simulink model "fourteen_bus_partial_linear"  (R2020b)
settings: Solver=VariableStepAuto  StartTime=0.0  StopTime=1  RelTol=1e-3
libraries: powerlib x95, powerlib_meascontrol x2
(part 2 of 2)

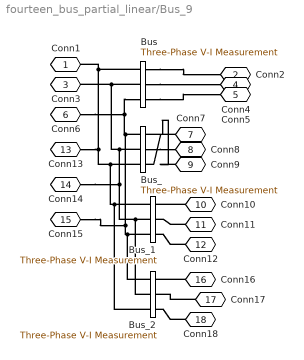
== system fourteen_bus_partial_linear/Bus_9 ==
  Bus : powerlib/Measurements/Three-Phase V-I Measurement  VoltageMeasurement=phase-to-phase  SetLabelV=on  LabelV=VB_9  Vpu=off  VpuLL=off  CurrentMeasurement=yes  SetLabelI=on  LabelI=IB_9  Ipu=off  Pbase=100e6  Vbase=500e3  OutputType=Complex  PhasorSimulation=off  PSBequivalent=0
  Bus_ : powerlib/Measurements/Three-Phase V-I Measurement  VoltageMeasurement=phase-to-phase  SetLabelV=on  LabelV=V_B9_9  Vpu=off  VpuLL=off  CurrentMeasurement=yes  SetLabelI=on  LabelI=I_B9_9  Ipu=off  Pbase=100e6  Vbase=500e3  OutputType=Complex  PhasorSimulation=off  PSBequivalent=0
  Bus_1 : powerlib/Measurements/Three-Phase V-I Measurement  VoltageMeasurement=phase-to-phase  SetLabelV=on  LabelV=V_B9  Vpu=off  VpuLL=off  CurrentMeasurement=yes  SetLabelI=on  LabelI=I_B9  Ipu=off  Pbase=100e6  Vbase=500e3  OutputType=Complex  PhasorSimulation=off  PSBequivalent=0
  Bus_2 : powerlib/Measurements/Three-Phase V-I Measurement  VoltageMeasurement=phase-to-phase  SetLabelV=on  LabelV=V_B9__9  Vpu=off  VpuLL=off  CurrentMeasurement=yes  SetLabelI=on  LabelI=I_B9__9  Ipu=off  Pbase=100e6  Vbase=500e3  OutputType=Complex  PhasorSimulation=off  PSBequivalent=0
  Conn1 : PMIOPort  Side=Left
  Conn2 : PMIOPort  Port=2  Side=Right
  Conn3 : PMIOPort  Port=3  Side=Left
  Conn4 : PMIOPort  Port=4  Side=Right
  Conn5 : PMIOPort  Port=5  Side=Right
  Conn6 : PMIOPort  Port=6  Side=Left
  Conn7 : PMIOPort  Port=7  Side=Right
  Conn8 : PMIOPort  Port=8  Side=Right
  Conn9 : PMIOPort  Port=9  Side=Right
  Conn10 : PMIOPort  Port=10  Side=Right
  Conn11 : PMIOPort  Port=11  Side=Right
  Conn12 : PMIOPort  Port=12  Side=Right
  Conn13 : PMIOPort  Port=13  Side=Left
  Conn14 : PMIOPort  Port=14  Side=Left
  Conn15 : PMIOPort  Port=15  Side=Left
  Conn16 : PMIOPort  Port=16  Side=Right
  Conn17 : PMIOPort  Port=17  Side=Right
  Conn18 : PMIOPort  Port=18  Side=Right
  connections:
  Bus/LConn1 -- Conn1/RConn1 -- Conn13/RConn1 -- Bus_/LConn3 -- Bus_1/LConn1 -- Bus_2/LConn3
  Conn3/RConn1 -- Bus/LConn2 -- Bus_/LConn2 -- Conn14/RConn1 -- Bus_1/LConn2 -- Bus_2/LConn2
  Bus_/RConn2 -- Conn8/RConn1
  Bus/RConn2 -- Conn4/RConn1
  Bus/LConn3 -- Conn6/RConn1 -- Bus_/LConn1 -- Conn15/RConn1 -- Bus_1/LConn3 -- Bus_2/LConn1
  Bus/RConn1 -- Conn2/RConn1
  Bus/RConn3 -- Conn5/RConn1
  Conn10/RConn1 -- Bus_1/RConn1
  Conn11/RConn1 -- Bus_1/RConn2
  Conn12/RConn1 -- Bus_1/RConn3
  Conn16/RConn1 -- Bus_2/RConn1
  Conn17/RConn1 -- Bus_2/RConn2
  Conn18/RConn1 -- Bus_2/RConn3
  Conn7/RConn1 -- Bus_/RConn3
  Conn9/RConn1 -- Bus_/RConn1

== system fourteen_bus_partial_linear/Subsystem ==
  Ia : Inport
  Ib : Inport  Port=2
  Ic : Inport  Port=3
  Controlled Current Source10 : powerlib/Electrical Sources/Controlled Current Source  Initialize=on  Source_Type=AC  Amplitude=0  Phase=0  Frequency=0  Measurements=None
  Controlled Current Source11 : powerlib/Electrical Sources/Controlled Current Source  Initialize=on  Source_Type=AC  Amplitude=0  Phase=0  Frequency=0  Measurements=None
  Controlled Current Source9 : powerlib/Electrical Sources/Controlled Current Source  Initialize=on  Source_Type=AC  Amplitude=0  Phase=0  Frequency=0  Measurements=None
  Ground2 : powerlib/Elements/Ground  LConnTagsString=a
  A : PMIOPort  Side=Right
  B : PMIOPort  Port=2  Side=Right
  C : PMIOPort  Port=3  Side=Right
  wires:
  Ia/1 -> Controlled Current Source9/1
  Ic/1 -> Controlled Current Source11/1
  Ib/1 -> Controlled Current Source10/1
  connections:
  Controlled Current Source10/RConn1 -- B/RConn1
  Controlled Current Source9/RConn1 -- A/RConn1
  Controlled Current Source11/RConn1 -- C/RConn1
  Controlled Current Source11/LConn1 -- Controlled Current Source9/LConn1 -- Controlled Current Source10/LConn1 -- Ground2/LConn1

== system fourteen_bus_partial_linear/Subsystem10 ==
  From Workspace15 : FromWorkspace  VariableName=load5_Ia_ts
  From Workspace16 : FromWorkspace  VariableName=load5_Ib_ts
  From Workspace17 : FromWorkspace  VariableName=load5_Ic_ts
  Subsystem3 : Subsystem
  A : PMIOPort  Side=Right
  B : PMIOPort  Port=2  Side=Right
  C : PMIOPort  Port=3  Side=Right
  wires:
  From Workspace15/1 -> Subsystem3/1(Ia)
  From Workspace17/1 -> Subsystem3/3(Ic)
  From Workspace16/1 -> Subsystem3/2(Ib)
  connections:
  Subsystem3/RConn2 -- B/RConn1
  Subsystem3/RConn1 -- A/RConn1
  Subsystem3/RConn3 -- C/RConn1

== system fourteen_bus_partial_linear/Subsystem11 ==
  From Workspace15 : FromWorkspace  VariableName=load2_Ia_ts
  From Workspace16 : FromWorkspace  VariableName=load2_Ib_ts
  From Workspace17 : FromWorkspace  VariableName=load2_Ic_ts
  Subsystem3 : Subsystem
  A : PMIOPort  Side=Right
  B : PMIOPort  Port=2  Side=Right
  C : PMIOPort  Port=3  Side=Right
  wires:
  From Workspace15/1 -> Subsystem3/1(Ia)
  From Workspace17/1 -> Subsystem3/3(Ic)
  From Workspace16/1 -> Subsystem3/2(Ib)
  connections:
  Subsystem3/RConn2 -- B/RConn1
  Subsystem3/RConn1 -- A/RConn1
  Subsystem3/RConn3 -- C/RConn1

== system fourteen_bus_partial_linear/Subsystem12 ==
  From Workspace10 : FromWorkspace  VariableName=sc3_Ib_ts
  From Workspace11 : FromWorkspace  VariableName=sc3_Ic_ts
  From Workspace9 : FromWorkspace  VariableName=sc3_Ia_ts
  Subsystem1 : Subsystem
  A : PMIOPort  Side=Right
  B : PMIOPort  Port=2  Side=Right
  C : PMIOPort  Port=3  Side=Right
  wires:
  From Workspace11/1 -> Subsystem1/3(Ic)
  From Workspace9/1 -> Subsystem1/1(Ia)
  From Workspace10/1 -> Subsystem1/2(Ib)
  connections:
  Subsystem1/RConn1 -- A/RConn1
  Subsystem1/RConn2 -- B/RConn1
  Subsystem1/RConn3 -- C/RConn1

== system fourteen_bus_partial_linear/Subsystem10/Subsystem3 ==
  Ia : Inport
  Ib : Inport  Port=2
  Ic : Inport  Port=3
  Controlled Current Source10 : powerlib/Electrical Sources/Controlled Current Source  Initialize=on  Source_Type=AC  Amplitude=0  Phase=0  Frequency=0  Measurements=None
  Controlled Current Source11 : powerlib/Electrical Sources/Controlled Current Source  Initialize=on  Source_Type=AC  Amplitude=0  Phase=0  Frequency=0  Measurements=None
  Controlled Current Source9 : powerlib/Electrical Sources/Controlled Current Source  Initialize=on  Source_Type=AC  Amplitude=0  Phase=0  Frequency=0  Measurements=None
  Ground2 : powerlib/Elements/Ground  LConnTagsString=a
  A : PMIOPort  Side=Right
  B : PMIOPort  Port=2  Side=Right
  C : PMIOPort  Port=3  Side=Right
  wires:
  Ia/1 -> Controlled Current Source9/1
  Ic/1 -> Controlled Current Source11/1
  Ib/1 -> Controlled Current Source10/1
  connections:
  Controlled Current Source10/RConn1 -- B/RConn1
  Controlled Current Source9/RConn1 -- A/RConn1
  Controlled Current Source11/RConn1 -- C/RConn1
  Controlled Current Source10/LConn1 -- Controlled Current Source11/LConn1 -- Controlled Current Source9/LConn1 -- Ground2/LConn1

== system fourteen_bus_partial_linear/Subsystem11/Subsystem3 ==
  Ia : Inport
  Ib : Inport  Port=2
  Ic : Inport  Port=3
  Controlled Current Source10 : powerlib/Electrical Sources/Controlled Current Source  Initialize=on  Source_Type=AC  Amplitude=0  Phase=0  Frequency=0  Measurements=None
  Controlled Current Source11 : powerlib/Electrical Sources/Controlled Current Source  Initialize=on  Source_Type=AC  Amplitude=0  Phase=0  Frequency=0  Measurements=None
  Controlled Current Source9 : powerlib/Electrical Sources/Controlled Current Source  Initialize=on  Source_Type=AC  Amplitude=0  Phase=0  Frequency=0  Measurements=None
  Ground2 : powerlib/Elements/Ground  LConnTagsString=a
  A : PMIOPort  Side=Right
  B : PMIOPort  Port=2  Side=Right
  C : PMIOPort  Port=3  Side=Right
  wires:
  Ia/1 -> Controlled Current Source9/1
  Ic/1 -> Controlled Current Source11/1
  Ib/1 -> Controlled Current Source10/1
  connections:
  Controlled Current Source10/RConn1 -- B/RConn1
  Controlled Current Source9/RConn1 -- A/RConn1
  Controlled Current Source11/RConn1 -- C/RConn1
  Controlled Current Source10/LConn1 -- Controlled Current Source11/LConn1 -- Controlled Current Source9/LConn1 -- Ground2/LConn1

== system fourteen_bus_partial_linear/Subsystem12/Subsystem1 ==
  Ia : Inport
  Ib : Inport  Port=2
  Ic : Inport  Port=3
  Controlled Current Source10 : powerlib/Electrical Sources/Controlled Current Source  Initialize=on  Source_Type=AC  Amplitude=0  Phase=0  Frequency=0  Measurements=None
  Controlled Current Source11 : powerlib/Electrical Sources/Controlled Current Source  Initialize=on  Source_Type=AC  Amplitude=0  Phase=0  Frequency=0  Measurements=None
  Controlled Current Source9 : powerlib/Electrical Sources/Controlled Current Source  Initialize=on  Source_Type=AC  Amplitude=0  Phase=0  Frequency=0  Measurements=None
  Ground2 : powerlib/Elements/Ground  LConnTagsString=a
  A : PMIOPort  Side=Right
  B : PMIOPort  Port=2  Side=Right
  C : PMIOPort  Port=3  Side=Right
  wires:
  Ia/1 -> Controlled Current Source9/1
  Ic/1 -> Controlled Current Source11/1
  Ib/1 -> Controlled Current Source10/1
  connections:
  Controlled Current Source10/RConn1 -- B/RConn1
  Controlled Current Source9/RConn1 -- A/RConn1
  Controlled Current Source11/RConn1 -- C/RConn1
  Controlled Current Source11/LConn1 -- Ground2/LConn1 -- Controlled Current Source10/LConn1 -- Controlled Current Source9/LConn1
